simulink model "lqrVsNlin_115"  (Simulink 7.9)
settings: Solver=ode45  StartTime=0.0  StopTime=10.0  RelTol=1e-3
values from neighbouring files (symbols this model uses):
  AMin = [ ... (first row only)    [LqrObs1_15.m]
  Aoss = AMin-L*ClocalMin    [LqrObs1_15.m]
  BMin = [ ... (first row only)    [LqrObs1_15.m]
  Boss = [BMin-L*D L]    [LqrObs1_15.m]
  ClocalMin = [ ... (first row only)    [LqrObs1_15.m]
  Coss = eye(size(AMin))    [LqrObs1_15.m]
  D = zeros(4,4)    [LqrObs1_15.m]
  Doss = zeros(size(Boss))    [LqrObs1_15.m]
  g = 9.81    [LqrObs1_15.m]
  If = -0.3559    [LqrObs1_15.m]
  K = lqr(AMin,BMin,Qie,Rie)    [LqrObs1_15.m]
  mq = 1.20    (= 1.2)    [LqrObs1_15.m]
  refs = [-3 0 0 0 45 0 0 0 ]    [LqrObs1_15.m]
libraries: simulink_extras x4, aerolib6dof2 x1
settings Model: Creator=UserK  LastModifiedBy=userk
settings DataIOCC: SignalLoggingSaveFormat=Dataset
settings OptimizationCC: ExpressionDepthLimit=128
settings DebuggingCC: UnderspecifiedInitializationDetection=Simplified  MergeDetectMultiDrivingBlocksExec=error  SolverPrmCheckMsg=none  FrameProcessingCompatibilityMsg=error  StateNameClashWarn=none
settings CodeAppCC: CustomSymbolStrType=$N$R$M_T
settings GRTTargetCC: CodeReplacementLibrary=None  CPPClassGenCompliant=on

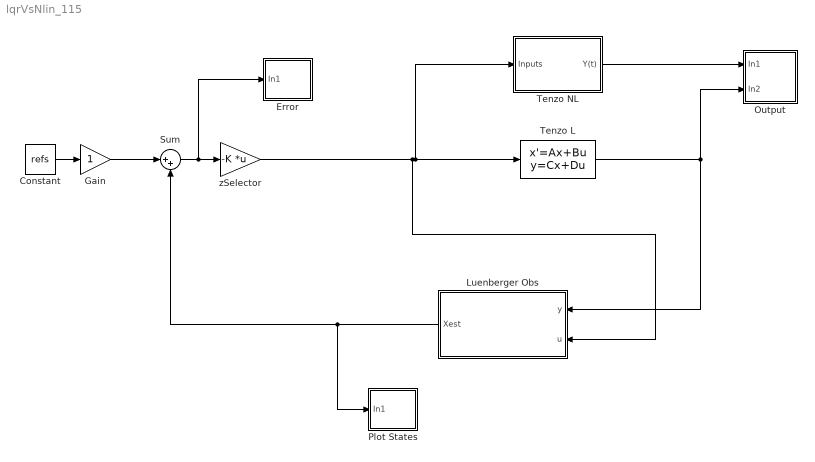
== system lqrVsNlin_115 ==
  Constant : Constant  Value=refs
  Error : Subsystem
  Gain : Gain
  Luenberger Obs : Subsystem
  Output : Subsystem
  Plot States : Subsystem
  Sum : Sum  Inputs=|++
  Tenzo L : StateSpace  A=AMin  B=BMin  C=ClocalMin  D=D  X0=[20 0 45 0 180 0 0 0 ]
  Tenzo NL : Subsystem
  zSelector : Gain  Gain=-K  Multiplication=Matrix(K*u)
  wires:
  Tenzo L/1 -> Luenberger Obs/1(y), Output/2(In2)
  Luenberger Obs/1(Xest) -> Plot States/1(In1), Sum/2
  Constant/1 -> Gain/1
  Gain/1 -> Sum/1
  Sum/1 -> Error/1(In1), zSelector/1
  zSelector/1 -> Luenberger Obs/2(u), Tenzo L/1, Tenzo NL/1(Inputs)
  Tenzo NL/1(Y(t)) -> Output/1(In1)

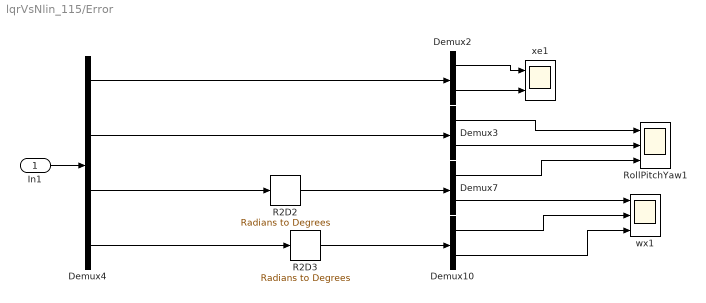
== system lqrVsNlin_115/Error ==
  In1 : Inport
  Demux{2..3,7,10} (4 alike) : Demux  Outputs=2
  Demux4 : Demux
  R2D2 : simulink_extras/Transformations/Radians to Degrees
  R2D3 : simulink_extras/Transformations/Radians to Degrees
  RollPitchYaw1 : Scope  NumInputPorts=3
      settings: YMin=-5~-5~-5  YMax=5~5~5  SaveName=ScopeData21
  wx1 : Scope  NumInputPorts=3
      settings: TimeRange=15  YMin=-5~-5~-5  YMax=5~5~5  SaveName=ScopeData24
  xe1 : Scope  NumInputPorts=2
      settings: TimeRange=3  YMin=1.6e-05~1.6e-05  YMax=3e-05~3e-05  SaveName=ScopeData25
  wires:
  Demux3/1 -> RollPitchYaw1/1
  Demux3/2 -> RollPitchYaw1/2
  Demux7/1 -> RollPitchYaw1/3
  Demux7/2 -> wx1/1
  Demux10/1 -> wx1/2
  Demux10/2 -> wx1/3
  In1/1 -> Demux4/1
  Demux4/3 -> R2D2/1
  R2D3/1 -> Demux10/1
  R2D2/1 -> Demux7/1
  Demux2/2 -> xe1/2
  Demux2/1 -> xe1/1
  Demux4/4 -> R2D3/1
  Demux4/2 -> Demux3/1
  Demux4/1 -> Demux2/1

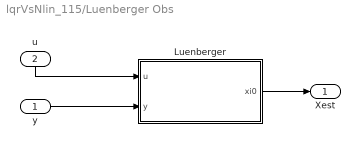
== system lqrVsNlin_115/Luenberger Obs ==
  y : Inport
  u : Inport  Port=2
  Luenberger : Subsystem
  Xest : Outport
  wires:
  Luenberger/1(xi0) -> Xest/1
  u/1 -> Luenberger/1(u)
  y/1 -> Luenberger/2(y)

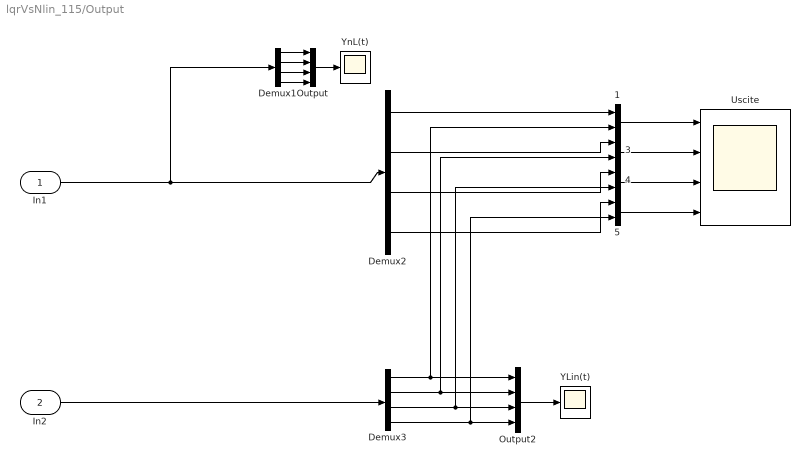
== system lqrVsNlin_115/Output ==
  In1 : Inport
  In2 : Inport  Port=2
  {1,3..5} (4 alike) : Concatenate
  Demux1 : Demux
  Demux2 : Demux
  Demux3 : Demux
  Output : Concatenate  NumInputs=4
  Output2 : Concatenate  NumInputs=4
  Uscite : Scope  NumInputPorts=4
      settings: YMin=2500~-5~-5~-5  YMax=7000~5~5~5
  YLin(t) : Scope
      settings: YMin=2500  YMax=7000
  YnL(t) : Scope
      settings: YMin=2500  YMax=7000  SaveName=ScopeData20
  wires:
  In1/1 -> Demux2/1, Demux1/1
  In2/1 -> Demux3/1
  Demux2/1 -> 1/1
  Output2/1 -> YLin(t)/1
  Demux3/1 -> Output2/1, 1/2
  Demux3/2 -> Output2/2, 3/2
  Demux3/3 -> Output2/3, 4/2
  Demux3/4 -> Output2/4, 5/2
  1/1 -> Uscite/1
  3/1 -> Uscite/2
  4/1 -> Uscite/3
  5/1 -> Uscite/4
  Demux2/2 -> 3/1
  Demux2/3 -> 4/1
  Demux2/4 -> 5/1
  Demux1/4 -> Output/4
  Demux1/3 -> Output/3
  Demux1/1 -> Output/1
  Demux1/2 -> Output/2
  Output/1 -> YnL(t)/1

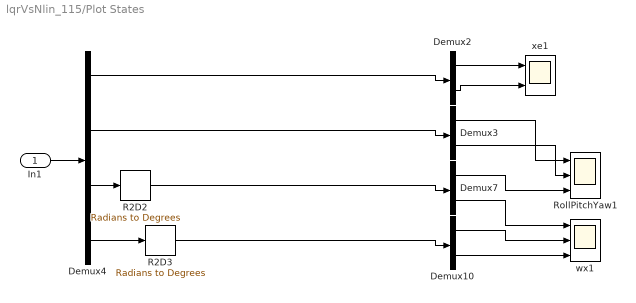
== system lqrVsNlin_115/Plot States ==
  In1 : Inport
  Demux{2..3,7,10} (4 alike) : Demux  Outputs=2
  Demux4 : Demux
  R2D2 : simulink_extras/Transformations/Radians to Degrees
  R2D3 : simulink_extras/Transformations/Radians to Degrees
  RollPitchYaw1 : Scope  NumInputPorts=3
      settings: YMin=-5~-5~-5  YMax=5~5~5  SaveName=ScopeData21
  wx1 : Scope  NumInputPorts=3
      settings: TimeRange=15  YMin=-5~-5~-5  YMax=5~5~5  SaveName=ScopeData24
  xe1 : Scope  NumInputPorts=2
      settings: TimeRange=3  YMin=1.6e-05~1.6e-05  YMax=3e-05~3e-05  SaveName=ScopeData25
  wires:
  Demux4/1 -> Demux2/1
  Demux4/2 -> Demux3/1
  Demux4/4 -> R2D3/1
  Demux2/1 -> xe1/1
  Demux2/2 -> xe1/2
  R2D2/1 -> Demux7/1
  R2D3/1 -> Demux10/1
  Demux4/3 -> R2D2/1
  In1/1 -> Demux4/1
  Demux10/2 -> wx1/3
  Demux10/1 -> wx1/2
  Demux7/2 -> wx1/1
  Demux7/1 -> RollPitchYaw1/3
  Demux3/2 -> RollPitchYaw1/2
  Demux3/1 -> RollPitchYaw1/1

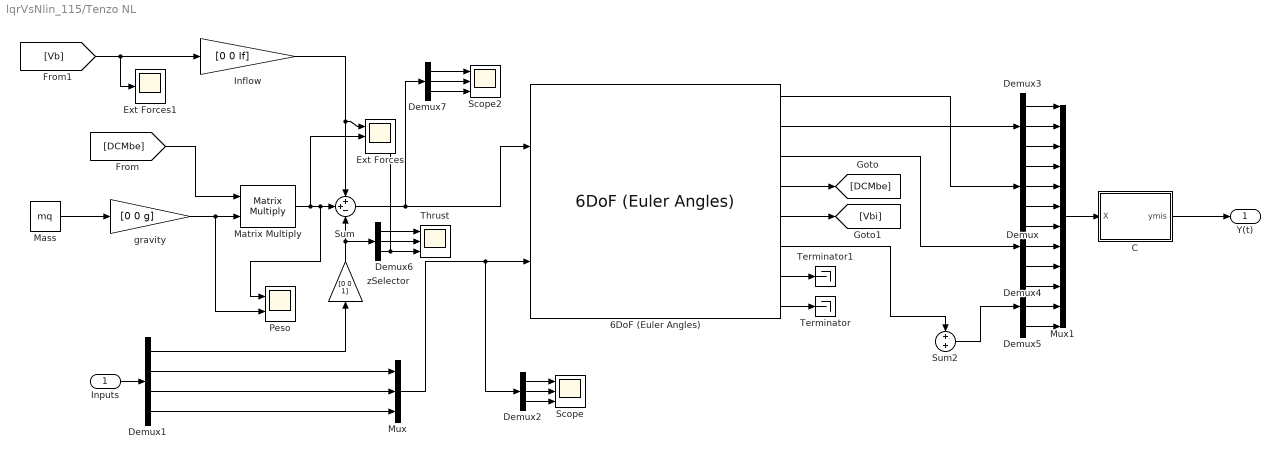
== system lqrVsNlin_115/Tenzo NL ==
  Inputs : Inport
  6DoF (Euler Angles) : aerolib6dof2/6DoF (Euler Angles)  units=Metric (MKS)  mtype=Fixed  rep=Euler Angles  xme_0=[0 0 0]  Vm_0=[0 0 0]  eul_0=[0 0 0]  pm_0=[0 0 0]  mass_0=mq  mass_e=0.5  mass_f=2.0  inertia=II  inertia_e=eye(3)  inertia_f=2*eye(3)  k_quat=1.0
  C : MATLAB Function  TreatAsAtomicUnit=on
  Demux{,2..7} (7 alike) : Demux  Outputs=3
  Demux1 : Demux
  Ext Forces : Scope  NumInputPorts=3
      settings: TimeRange=30  YMin=-950000~-8~-5  YMax=0~2~5  SaveName=ScopeData5  SampleInput=on  SampleTime=0.01
  Ext Forces1 : Scope
      settings: TimeRange=30  YMin=-950000  YMax=0  SaveName=ScopeData27  SampleInput=on  SampleTime=0.01
  Inflow : Gain  Gain=[0 0 If]
  Mass : Constant  Value=mq
  Matrix Multiply : Product  Multiplication=Matrix(*)
  Mux : Mux  Inputs=3
  Mux1 : Mux  Inputs=12
  Peso : Scope  NumInputPorts=2
      settings: TimeRange=30  YMin=-8~0  YMax=2~8.5  SaveName=ScopeData8  SampleInput=on  SampleTime=0.01
  Scope : Scope  NumInputPorts=3
      settings: YMin=26050.4~-1~-671.375  YMax=28792.6~1~-607.435  SaveName=ScopeData4
  Scope2 : Scope  NumInputPorts=3
      settings: YMin=-1~-1~-2.3  YMax=1~1~-0.4  SaveName=ScopeData23
  Sum : Sum  Inputs=++-
  Sum2 : Sum
  Terminator : Terminator
  Terminator1 : Terminator
  Thrust : Scope  NumInputPorts=3
      settings: YMin=-1~-1~-2.3  YMax=1~1~-0.4  SaveName=ScopeData7
  gravity : Gain  Gain=[0 0 g]
  zSelector : Gain  Gain=[0 0 1]
  Y(t) : Outport
  wires:
  6DoF (Euler Angles)/4 -> [DCMbe]
  [DCMbe] -> Matrix Multiply/1
  Mass/1 -> gravity/1
  gravity/1 -> Matrix Multiply/2, Peso/2
  Matrix Multiply/1 -> Sum/2, Peso/1, Ext Forces/2
  6DoF (Euler Angles)/5 -> [Vbi]
  [Vb] -> Inflow/1, Ext Forces1/1
  Inflow/1 -> Sum/1, Ext Forces/1
  Demux1/1 -> zSelector/1
  Demux1/2 -> Mux/1
  Demux1/3 -> Mux/2
  Demux1/4 -> Mux/3
  Sum/1 -> Demux7/1, 6DoF (Euler Angles)/1
  Mux/1 -> 6DoF (Euler Angles)/2, Demux2/1
  6DoF (Euler Angles)/1 -> Demux/1
  6DoF (Euler Angles)/2 -> Demux3/1
  Demux3/1 -> Mux1/1
  Demux3/2 -> Mux1/2
  Demux3/3 -> Mux1/3
  Demux/1 -> Mux1/4
  Demux/2 -> Mux1/5
  Demux/3 -> Mux1/6
  Demux4/1 -> Mux1/7
  Demux4/2 -> Mux1/8
  Demux4/3 -> Mux1/9
  Demux5/1 -> Mux1/10
  Demux5/2 -> Mux1/11
  Demux5/3 -> Mux1/12
  6DoF (Euler Angles)/8 -> Terminator/1
  6DoF (Euler Angles)/7 -> Terminator1/1
  6DoF (Euler Angles)/3 -> Demux4/1
  Inputs/1 -> Demux1/1
  Demux2/1 -> Scope/1
  Demux2/2 -> Scope/2
  Demux2/3 -> Scope/3
  Demux7/1 -> Scope2/1
  Demux7/2 -> Scope2/2
  Demux7/3 -> Scope2/3
  zSelector/1 -> Sum/3, Demux6/1
  Demux6/1 -> Thrust/1
  Demux6/2 -> Thrust/2
  Demux6/3 -> Thrust/3, Ext Forces/3
  6DoF (Euler Angles)/6 -> Sum2/1
  Sum2/1 -> Demux5/1
  Mux1/1 -> C/1(X)
  C/1(ymis) -> Y(t)/1

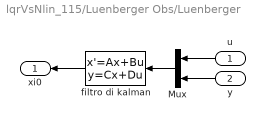
== system lqrVsNlin_115/Luenberger Obs/Luenberger ==
  u : Inport
  y : Inport  Port=2
  Mux : Mux  Inputs=[4 4]
  filtro di kalman : StateSpace  A=Aoss  B=Boss  C=Coss  D=Doss  X0=[0 0 0 0 0 0 0 0]
  xi0 : Outport
  wires:
  Mux/1 -> filtro di kalman/1
  u/1 -> Mux/1
  filtro di kalman/1 -> xi0/1
  y/1 -> Mux/2

== matlab function Tenzo NL/C ==
  data: X input double; ymis output double
function ymis = fcn(X)
%#codegen

Cmis = [0 0 0 0 0 0 1 0 0 0 0 0;
        0 0 0 0 0 0 0 1 0 0 0 0;
        0 0 0 0 0 0 0 0 1 0 0 0;
        0 0 1 0 0 0 0 0 0 0 0 0];
ymis = Cmis*X;
